simulink model "problem_1"  (R2020b)
settings: Solver=VariableStepAuto  StartTime=0.0  StopTime=10  MaxStep=0.01  RelTol=1e-3
PreLoadFcn:
  | vars
values from neighbouring files (symbols this model uses):
  b = 50    [vars.m]
  k1 = 50    [vars.m]
  k12 = 2    [vars.m]
  m1 = 100    [vars.m]
  m2 = 0.9    [vars.m]
settings Model: Creator=hp  LastModifiedBy=hp

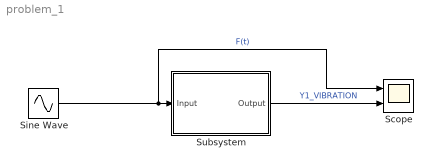
== system problem_1 ==
  Scope : Scope  NumInputPorts=2
  Sine Wave : Sin  Amplitude=2  Frequency=10  SampleTime=0
  Subsystem : Subsystem
  wires:
  Sine Wave/1 -> Scope/1, Subsystem/1(Input)  "F(t)"
  Subsystem/1(Output) -> Scope/2  "Y1_VIBRATION"

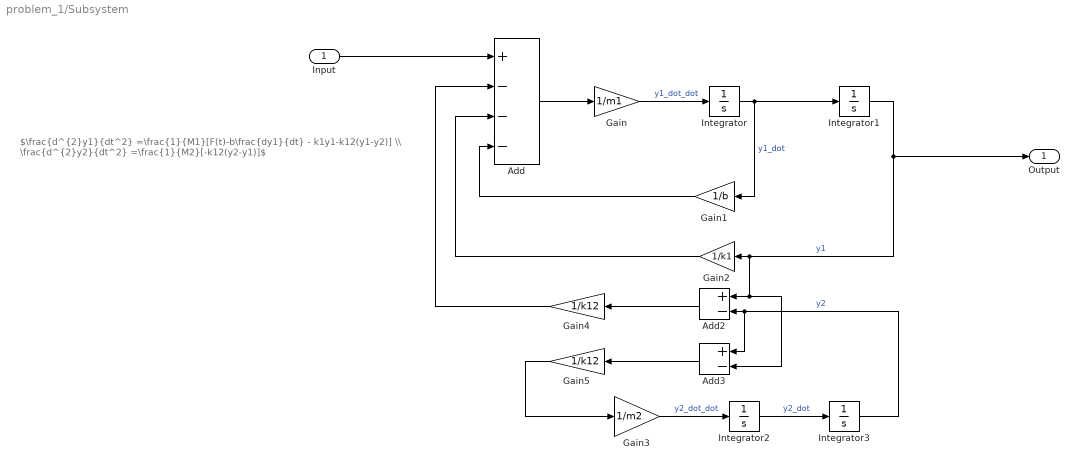
== system problem_1/Subsystem ==
  note: $\frac{d^{2}y1}{dt^2} =\frac{1}{M1}[F(t)-b\frac{dy1}{dt} - k1y1-k12(y1-y2)] \\ \frac{d^{2}y2}{dt^2} =\frac{1}{M2}[-k12(y2-y1)]$
  Input : Inport
  Add : Sum  Inputs=+---
  Add2 : Sum  Inputs=+-
  Add3 : Sum  Inputs=+-
  Gain : Gain  Gain=1/m1
  Gain1 : Gain  Gain=1/b
  Gain2 : Gain  Gain=1/k1
  Gain3 : Gain  Gain=1/m2
  Gain4 : Gain  Gain=1/k12
  Gain5 : Gain  Gain=1/k12
  Integrator{,1..3} (4 alike) : Integrator
  Output : Outport
  wires:
  Gain/1 -> Integrator/1  "y1_dot_dot"
  Add/1 -> Gain/1
  Integrator1/1 -> Output/1, Add2/1, Add3/2, Gain2/1  "y1"
  Integrator/1 -> Gain1/1, Integrator1/1  "y1_dot"
  Gain5/1 -> Gain3/1
  Gain2/1 -> Add/3
  Input/1 -> Add/1
  Integrator3/1 -> Add3/1, Add2/2  "y2"
  Integrator2/1 -> Integrator3/1  "y2_dot"
  Add2/1 -> Gain4/1
  Gain3/1 -> Integrator2/1  "y2_dot_dot"
  Gain4/1 -> Add/2
  Gain1/1 -> Add/4
  Add3/1 -> Gain5/1
